simulink model "modeloPreditivo2"  (R2018b)
settings: Solver=VariableStepAuto  StartTime=0.0  StopTime=100  RelTol=1e-3
values from neighbouring files (symbols this model uses):
  A = [0 1 0 0 ... (first row only)    [dadosBallBeam.m]    (also in dadosTanqueQuatro.m = [-1/T1 0 A3/(A1*T3) 0; tanqueQuatroLinearizacao.m = double(subs(As,{h1,h2,h3,h4,v1,v2},{h10,h20,h30,h40,v10,v20})
  B = [0 0 0 1]'    [dadosBallBeam.m]    (also in dadosTanqueQuatro.m = [(y1*k1)/A1 0; tanqueQuatroLinearizacao.m = double(subs(Bs,{h1,h2,h3,h4,v1,v2},{h10,h20,h30,h40,v10,v20})
  C = [1 0 0 0]    [dadosBallBeam.m]    (also in dadosTanqueQuatro.m = [1 0 0 0; tanqueQuatroLinearizacao.m = [1 0 0 0)
  D = [0]    [dadosBallBeam.m]    (also in dadosTanqueQuatro.m = [0 0; tanqueQuatroLinearizacao.m = [0 0)
  h = 0.1    [MPC_sem_restricao.m]
undefined symbols (not defined in the file or in its folder): DiscIntNeverNeededParam, var
libraries: simulink x1
settings Model: Creator=Caléo  LastModifiedBy=Caléo

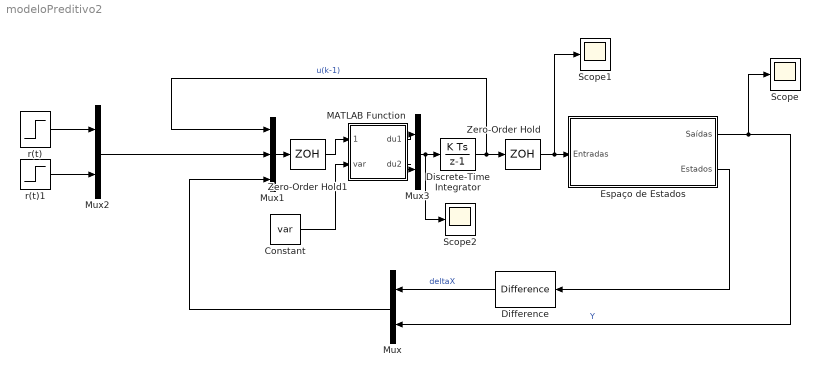
== system modeloPreditivo2 ==
  Constant : Constant  Value=var  OutDataTypeStr=Bus: var_bus
  Difference : simulink/Discrete/Difference  ICPrevInput=0.0  OutMin=[]  OutMax=[]  OutDataType=fixdt(1, 16)  OutScaling=2^-10  DoSatur=off
  Discrete-Time Integrator : DiscreteIntegrator  SampleTime=-1  ICPrevOutput=DiscIntNeverNeededParam  ICPrevScaledInput=DiscIntNeverNeededParam
  Espaço de Estados : Subsystem
  MATLAB Function : MATLAB Function  TreatAsAtomicUnit=on
  Mux : Mux  Inputs=2
  Mux1 : Mux  Inputs=3
  Mux2 : Mux  Inputs=2
  Mux3 : Mux  Inputs=2
  Scope : Scope
  Scope1 : Scope
  Scope2 : Scope
  Zero-Order Hold : ZeroOrderHold  SampleTime=h
  Zero-Order Hold1 : ZeroOrderHold  SampleTime=h
  r(t) : Step  Time=0  After=2  SampleTime=0
  r(t)1 : Step  Time=0  After=-0.5  SampleTime=0
  wires:
  Espaço de Estados/1(Saídas) -> Scope/1, Mux/2  "Y"
  Difference/1 -> Mux/1  "deltaX"
  Espaço de Estados/2(Estados) -> Difference/1
  Mux/1 -> Mux1/3
  Zero-Order Hold/1 -> Scope1/1, Espaço de Estados/1(Entradas)
  Discrete-Time Integrator/1 -> Mux1/1, Zero-Order Hold/1  "u(k-1)"
  r(t)/1 -> Mux2/1
  r(t)1/1 -> Mux2/2
  Mux2/1 -> Mux1/2
  Mux1/1 -> Zero-Order Hold1/1
  Zero-Order Hold1/1 -> MATLAB Function/1(entrada)
  Mux3/1 -> Scope2/1, Discrete-Time Integrator/1
  Constant/1 -> MATLAB Function/2(var)
  MATLAB Function/1(du1) -> Mux3/1
  MATLAB Function/2(du2) -> Mux3/2

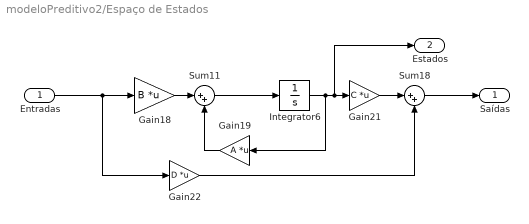
== system modeloPreditivo2/Espaço de Estados ==
  Entradas : Inport
  Gain18 : Gain  Gain=B  Multiplication=Matrix(K*u)
  Gain19 : Gain  Gain=A  Multiplication=Matrix(K*u)
  Gain21 : Gain  Gain=C  Multiplication=Matrix(K*u)
  Gain22 : Gain  Gain=D  Multiplication=Matrix(K*u)
  Integrator6 : Integrator
  Sum11 : Sum  Inputs=|++
  Sum18 : Sum  Inputs=|++
  Saídas : Outport
  Estados : Outport  Port=2
  wires:
  Entradas/1 -> Gain22/1, Gain18/1
  Sum18/1 -> Saídas/1
  Gain22/1 -> Sum18/2
  Gain18/1 -> Sum11/1
  Gain19/1 -> Sum11/2
  Integrator6/1 -> Gain19/1, Estados/1, Gain21/1
  Sum11/1 -> Integrator6/1
  Gain21/1 -> Sum18/1

== matlab function modeloPreditivo2/MATLAB Function ==
  data: entrada input; du1 output; du2 output; var input
function [du1,du2]  = MPC_com_restricao(entrada,var)
%#codegen
du1 = 0;
du2 = 0;

coder.extrinsic('quadprog');
[N,Nu,Bp,Cp,Qp,Rp,Ap,Ya,Yb,Ua,Ub,M,Dua,Dub] = deal(var.N,var.Nu,var.Bp,var.Cp,var.Qp,var.Rp,var.Ap,var.Ya,var.Yb,var.Ua,var.Ub,var.M,var.Dua,var.Dub);

up = entrada(1:2);
w = entrada(3:4);
Xk = entrada(5:end);


W = repmat(w,N,1);
H = 2*(Bp'*Cp'*Qp*Cp*Bp + Rp);
f = 2*(Qp*Cp*Bp)'*(Cp*Ap*Xk - W);

Um = repmat(up,Nu,1);


Ra = [Ya*Cp*Bp;Ua*M;Dua];
Rb = [Yb-Ya*Cp*Ap*Xk;Ub-Ua*Um;Dub];
% Ra = [Ya*Cp*Bp;Dua];
% Rb = [Yb-Ya*Cp*Ap*Xk;Dub];
du = quadprog(H,f,Ra,Rb);

du1 = du(1);
du2 = du(2);
end
